simulink model "OpenLoop_NonLin"  (Simulink 7.9)
settings: Solver=ode45  StartTime=0.0  StopTime=100  RelTol=1e-3
settings Model: Creator=mchi9aa4  LastModifiedBy=mchi9aa4
settings DataIOCC: Refine=10

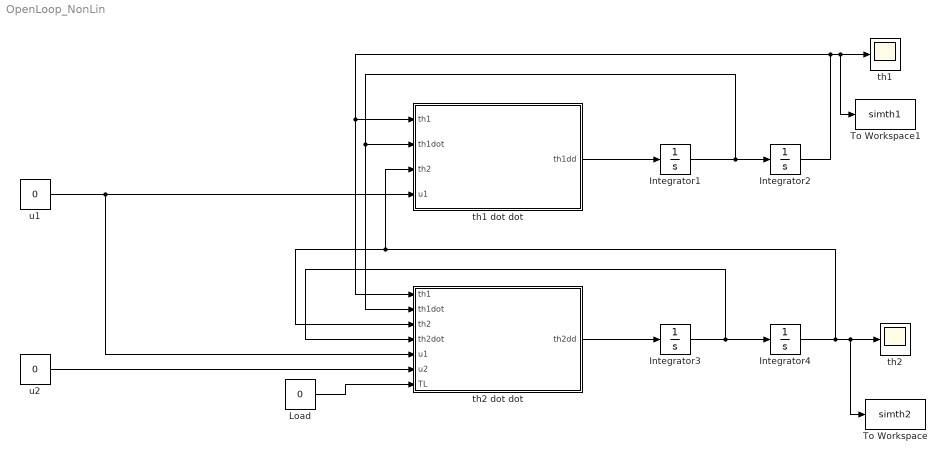
== system OpenLoop_NonLin ==
  Integrator1 : Integrator
  Integrator2 : Integrator  InitialCondition=pi/2.1
  Integrator3 : Integrator
  Integrator4 : Integrator
  Load : Constant  Value=0
  To Workspace : ToWorkspace  VariableName=simth2  SampleTime=-1
  To Workspace1 : ToWorkspace  VariableName=simth1  SampleTime=-1
  th1 : Scope
  th1 dot dot : MATLAB Function  TreatAsAtomicUnit=on
  th2 : Scope
  th2 dot dot : MATLAB Function  TreatAsAtomicUnit=on
  u1 : Constant  Value=0
  u2 : Constant  Value=0
  wires:
  th1 dot dot/1(th1dd) -> Integrator1/1
  Integrator1/1 -> Integrator2/1, th1 dot dot/2(th1dot), th2 dot dot/2(th1dot)
  th2 dot dot/1(th2dd) -> Integrator3/1
  Integrator3/1 -> Integrator4/1, th2 dot dot/4(th2dot)
  Integrator2/1 -> th2 dot dot/1(th1), th1 dot dot/1(th1), th1/1, To Workspace1/1
  Integrator4/1 -> th2 dot dot/3(th2), th1 dot dot/3(th2), th2/1, To Workspace/1
  Load/1 -> th2 dot dot/7(TL)
  u2/1 -> th2 dot dot/6(u2)
  u1/1 -> th1 dot dot/4(u1), th2 dot dot/5(u1)

== matlab function th2 dot dot ==
  data: th1 input double; th1dot input double; th2 input double; th2dd output double; th2dot input double; u1 input double; u2 input double; TL input double
function th2dd = fcn(th1, th1dot, th2, th2dot, u1, u2, TL)
%#codegen

th2dotdot = (75*u2)/8 - (75*th2dot)/8 - (75*TL)/8 - (75*cos(th1 + th2))/2 + (8*cos(th1))/((16*cos(th2))/25 + 76/75) + th1dot/(4*((8*cos(th2))/25 + 38/75)) - u1/(2*((8*cos(th2))/25 + 38/75)) + (20*cos(th1 + asin(sin(th2)/(5*((4*cos(th2))/25 + 1/5)^(1/2))))*((4*cos(th2))/25 + 1/5)^(1/2))/((8*cos(th2))/25 + 38/75);

th2dd = th2dotdot;

== matlab function th1 dot dot ==
  data: th1 input double; th1dot input double; th2 input double; th1dd output double; u1 input double
function th1dd = fcn(th1, th1dot, th2, u1)
%#codegen

th1dotdot = u1/(2*((8*cos(th2))/25 + 38/75)) - th1dot/(4*((8*cos(th2))/25 + 38/75)) - (8*cos(th1))/((16*cos(th2))/25 + 76/75) - (20*cos(th1 + asin(sin(th2)/(5*((4*cos(th2))/25 + 1/5)^(1/2))))*((4*cos(th2))/25 + 1/5)^(1/2))/((8*cos(th2))/25 + 38/75);

th1dd = th1dotdot;
